simulink model "Detumble_Sim"  (R2020a)
settings: Solver=ode4  StartTime=0.0  StopTime=10  FixedStep=0.01  RelTol=1e-3  EnableMultiTasking=on
values from neighbouring files (symbols this model uses):
  E_b_ECI = [phi_b_ECI; theta_b_ECI; psi_b_ECI]    [Detumble_Initial.m]
  omega_b_ECI = [-0.05; 0.03; 0.2]    [Detumble_Initial.m]
  quat_b_ECI = [epsilon_b_ECI; eta_b_ECI]    [Detumble_Initial.m]
settings Model: SimulationMode=external  Creator=sheab  LastModifiedBy=sheab
settings SolverCC: ConcurrentTasks=on  AutoInsertRateTranBlk=on
settings DataIOCC: SaveFormat=StructureWithTime
settings OptimizationCC: BlockReduction=off  OptimizeBlockIOStorage=off
settings DebuggingCC: UnconnectedInputMsg=none  UnconnectedOutputMsg=none  UnconnectedLineMsg=none
settings HardwareCC: ProdBitPerPointer=32  ProdBitPerSizeT=32  ProdBitPerPtrDiffT=32  ProdLargestAtomicFloat=None  ProdWordSize=32  ProdLongLongMode=on  ProdHWDeviceType=Generic->32-bit x86 compatible
settings ModelReferenceCC: EnableRefExpFcnMdlSchedulingChecks=off
settings RTWCC: Description=Simulink Real-Time  SystemTargetFile=slrt.tlc  TemplateMakefile=slrt_default_tmf  CodeExecutionProfiling=on  RTWCompilerOptimization=on
settings SimulinkRealTimeCC: SupportVariableSizeSignals=on  RL32LogTETModifier=off  xPCConcurrentTasks=on

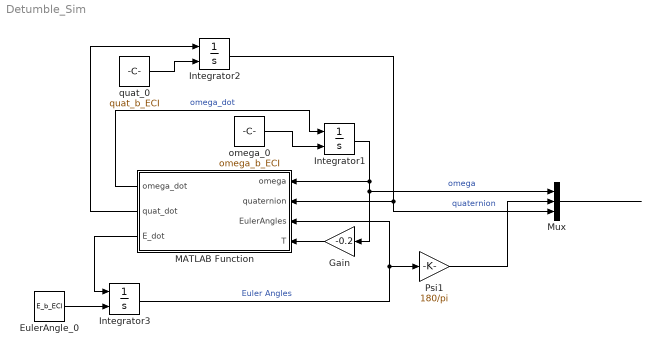
== system Detumble_Sim ==
  EulerAngle_0 : Constant  Value=E_b_ECI
  Gain : Gain  Gain=-0.2
  Integrator1 : Integrator  InitialConditionSource=external  InitialCondition=[.001,-.001,.002]
  Integrator2 : Integrator  InitialConditionSource=external  InitialCondition=[.001,-.001,.002]
  Integrator3 : Integrator  InitialConditionSource=external  InitialCondition=[.001,-.001,.002]
  MATLAB Function : MATLAB Function  TreatAsAtomicUnit=on
  Mux : Mux  Inputs=3
  Psi1 : Gain  Gain=180/pi
  omega_0 : Constant  Value=omega_b_ECI
  quat_0 : Constant  Value=quat_b_ECI
  wires:
  Gain/1 -> MATLAB Function/4(T)
  Integrator1/1 -> Mux/1, Gain/1, MATLAB Function/1(omega)  "omega"
  MATLAB Function/1(omega_dot) -> Integrator1/1  "omega_dot"
  omega_0/1 -> Integrator1/2
  MATLAB Function/2(quat_dot) -> Integrator2/1
  quat_0/1 -> Integrator2/2
  Integrator2/1 -> Mux/3, MATLAB Function/2(quaternion)  "quaternion"
  MATLAB Function/3(E_dot) -> Integrator3/1
  EulerAngle_0/1 -> Integrator3/2
  Integrator3/1 -> Psi1/1, MATLAB Function/3(EulerAngles)  "Euler Angles"
  Psi1/1 -> Mux/2
  Mux/1 -> ?

== matlab function Detumble_Sim/MATLAB Function ==
  data: omega input; quaternion input; EulerAngles input; omega_dot output; T input; quat_dot output; E_dot output
function [omega_dot, quat_dot, E_dot] = attitude2(omega, quaternion, EulerAngles, T)

% initial state
w = omega;
wx = [0, -w(3), w(2); w(3), 0, -w(1); -w(2), w(1), 0]; % epsilon cross

epsilon = quaternion(1:3,1);
epsilonx = [0, -epsilon(3), epsilon(2); epsilon(3), 0, -epsilon(1); -epsilon(2), epsilon(1), 0]; % epsilon cross
eta = quaternion(4,1);

phi = EulerAngles(1);
theta = EulerAngles(2);
psi = EulerAngles(3);

J = [426.6667, 0, 0; 0, 426.6667 , 0; 0, 0, 426.6667];

% derivatives
omega_dot = (J^(-1))*(T - wx*J*w);

epsilonp = 0.5*(eta*eye(3) + epsilonx)*w;
etap = -0.5*epsilon'*w; % derivative of eta
quat_dot = [epsilonp; etap];

Ep = [1, sin(phi)*tan(theta), cos(phi)*tan(theta); ...
          0, cos(phi), -sin(phi); ...
          0, sin(phi)*sec(theta), cos(phi)*sec(theta)];
E_dot = Ep*w;


end
